simulink model "sim_control_old_version"  (Simulink 10.2)
settings: Solver=ode45  StartTime=0.0  StopTime=Tsim  FixedStep=0.001  MaxStep=1e-4  RelTol=1e-3  EnableMultiTasking=on
values from neighbouring files (symbols this model uses):
  c = 2.76    [Question_8.m]    (also in call_sim.m; frf_fitting.m = param(2); gm_pm.m = 2.9123)
  eta = c/(2*m*w_n)    [Question_8.m]    (also in call_sim.m)
  k = 469    [Question_8.m]    (also in call_sim.m; frf_fitting.m = param(3); gm_pm.m = 451.39)
  Kd = Kd1(i)    [Question_8.m]    (also in call_sim.m = Kd; gm_pm.m = 0)
  Ki = Ki1(i)    [Question_8.m]    (also in call_sim.m = Ki; gm_pm.m = 0)
  Kp = Kp1(i)    [Question_8.m]    (also in call_sim.m = Kp; gm_pm.m = 2)
  m = 1.1    [Question_8.m]    (also in call_sim.m; frf_fitting.m = param(1); gm_pm.m = 0.8775)
  v0 = 0    [Question_8.m]    (also in call_sim.m)
  w_n = sqrt(k/m)    [Question_8.m]    (also in call_sim.m)
  x0 = 0    [Question_8.m]    (also in call_sim.m)
settings Model: Creator=snahata  LastModifiedBy=ymert
settings DataIOCC: LimitDataPoints=on
settings OptimizationCC: InitFltsAndDblsToZero=on
settings DebuggingCC: SaveWithParameterizedLinksMsg=none  SignalResolutionControl=TryResolveAllWithWarning  SolverPrmCheckMsg=warning  MultiTaskDSMMsg=warning  MultiTaskCondExecSysMsg=none  StateNameClashWarn=warning
settings GRTTargetCC: TargetFcnLib=ansi_tfl_tmw.mat

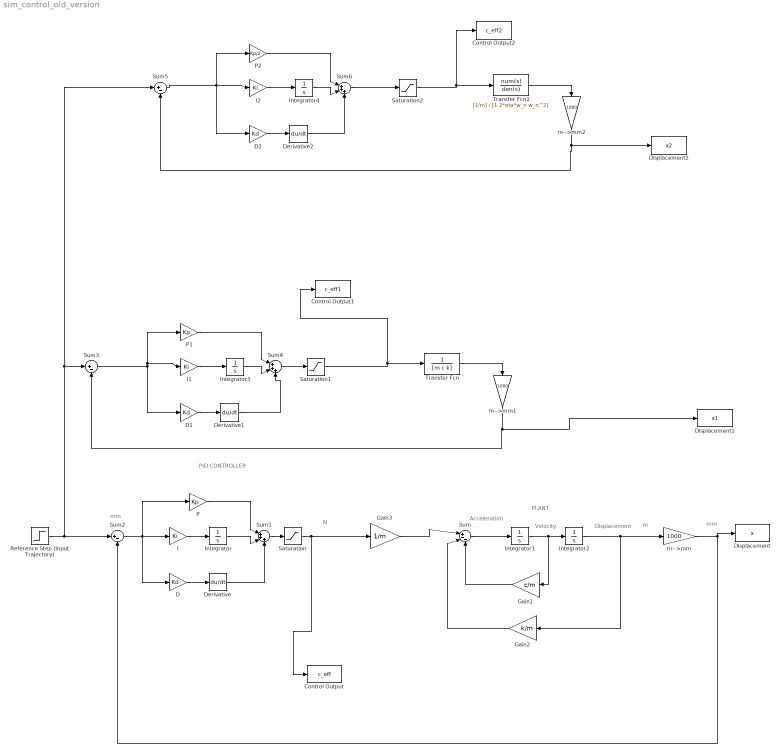
== system sim_control_old_version ==
  note: Acceleration
  note: Velocity
  note: Displacement
  note: mm
  note: N
  note: m
  note: mm
  note: PID CONTROLLER
  note: PLANT
  Control Output : ToWorkspace  VariableName=c_eff  SaveFormat=Timeseries  SampleTime=-1
  Control Output1 : ToWorkspace  VariableName=c_eff1  SaveFormat=Timeseries  SampleTime=-1
  Control Output2 : ToWorkspace  VariableName=c_eff2  SaveFormat=Timeseries  SampleTime=-1
  D : Gain  Gain=Kd
  D1 : Gain  Gain=Kd
  D2 : Gain  Gain=Kd
  Derivative : Derivative
  Derivative1 : Derivative
  Derivative2 : Derivative
  Displacement : ToWorkspace  VariableName=x  SaveFormat=Timeseries  SampleTime=-1
  Displacement1 : ToWorkspace  VariableName=x1  SaveFormat=Timeseries  SampleTime=-1
  Displacement2 : ToWorkspace  VariableName=x2  SaveFormat=Timeseries  SampleTime=-1
  Gain1 : Gain  Gain=c/m
  Gain2 : Gain  Gain=k/m
  Gain3 : Gain  Gain=1/m
  I : Gain  Gain=Ki
  I1 : Gain  Gain=Ki
  I2 : Gain  Gain=Ki
  Integrator : Integrator
  Integrator1 : Integrator  InitialCondition=v0
  Integrator2 : Integrator  InitialCondition=x0
  Integrator3 : Integrator
  Integrator4 : Integrator
  P : Gain  Gain=Kp
  P1 : Gain  Gain=Kp
  P2 : Gain  Gain=Kp/2
  Reference Step (Input Trajectory) : Step  After=3  SampleTime=0.01
  Saturation : Saturate  UpperLimit=15  LowerLimit=-15
  Saturation1 : Saturate  UpperLimit=15  LowerLimit=-15
  Saturation2 : Saturate  UpperLimit=15  LowerLimit=-15
  Sum : Sum  Inputs=|+--
  Sum1 : Sum  Inputs=|+++
  Sum2 : Sum  Inputs=|+-
  Sum3 : Sum  Inputs=|+-
  Sum4 : Sum  Inputs=|+++
  Sum5 : Sum  Inputs=|+-
  Sum6 : Sum  Inputs=|+++
  Transfer Fcn : TransferFcn  Denominator=[m c k]
  Transfer Fcn1 : TransferFcn  Numerator=[1/m]  Denominator=[1 2*eta*w_n w_n^2]
  m-->mm : Gain  Gain=1000
  m-->mm1 : Gain  Gain=1000
  m-->mm2 : Gain  Gain=1000
  wires:
  Sum/1 -> Integrator1/1
  Integrator1/1 -> Integrator2/1, Gain1/1
  Gain1/1 -> Sum/3
  Gain2/1 -> Sum/2
  Integrator2/1 -> Gain2/1, m-->mm/1
  D/1 -> Derivative/1
  I/1 -> Integrator/1
  Integrator/1 -> Sum1/2
  Derivative/1 -> Sum1/3
  P/1 -> Sum1/1
  Sum1/1 -> Saturation/1
  Sum2/1 -> D/1, I/1, P/1
  m-->mm/1 -> Displacement/1, Sum2/2
  Saturation/1 -> Control Output/1, Gain3/1
  Gain3/1 -> Sum/1
  Transfer Fcn/1 -> m-->mm1/1
  m-->mm1/1 -> Sum3/2, Displacement1/1
  Saturation1/1 -> Control Output1/1, Transfer Fcn/1
  Derivative1/1 -> Sum4/3
  Integrator3/1 -> Sum4/2
  P1/1 -> Sum4/1
  Sum4/1 -> Saturation1/1
  Sum3/1 -> I1/1, P1/1, D1/1
  I1/1 -> Integrator3/1
  D1/1 -> Derivative1/1
  I2/1 -> Integrator4/1
  D2/1 -> Derivative2/1
  P2/1 -> Sum6/1
  Derivative2/1 -> Sum6/3
  Sum6/1 -> Saturation2/1
  Transfer Fcn1/1 -> m-->mm2/1
  Saturation2/1 -> Control Output2/1, Transfer Fcn1/1
  Integrator4/1 -> Sum6/2
  Sum5/1 -> D2/1, I2/1, P2/1
  m-->mm2/1 -> Sum5/2, Displacement2/1
  Reference Step (Input Trajectory)/1 -> Sum5/1, Sum3/1, Sum2/1
